simulink model "Assignment4"  (R2014a)
settings: Solver=FixedStepDiscrete  StartTime=0.0  StopTime=10.0  FixedStep=1  RelTol=1e-3
libraries: simulink x20, hdlsllib x20
settings Model: Creator=vu.du  LastModifiedBy=vu.du

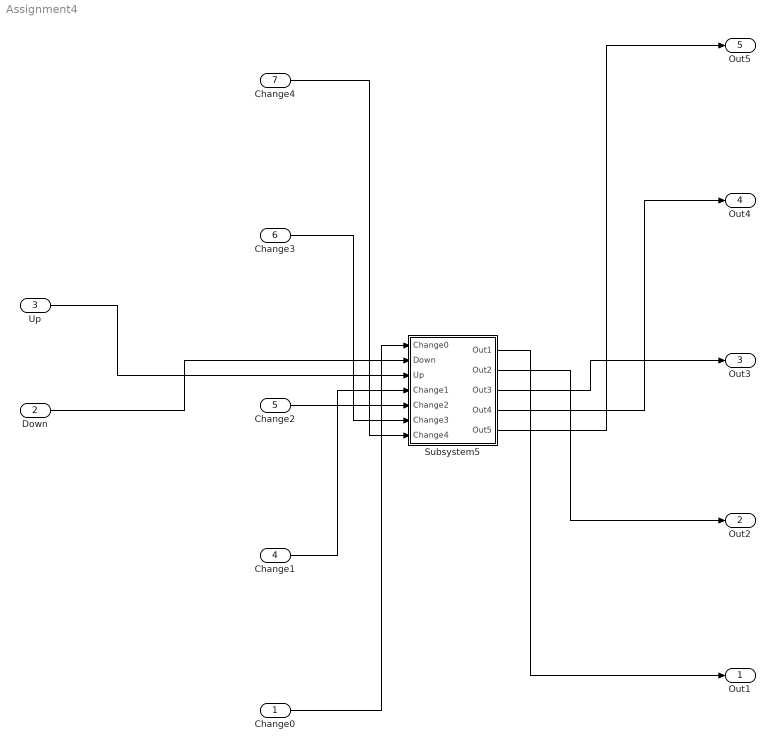
== system Assignment4 ==
  Change0 : Inport  OutDataTypeStr=boolean
  Down : Inport  Port=2  OutDataTypeStr=boolean
  Up : Inport  Port=3  OutDataTypeStr=boolean
  Change1 : Inport  Port=4  OutDataTypeStr=boolean
  Change2 : Inport  Port=5  OutDataTypeStr=boolean
  Change3 : Inport  Port=6  OutDataTypeStr=boolean
  Change4 : Inport  Port=7  OutDataTypeStr=boolean
  Subsystem5 : Subsystem  TreatAsAtomicUnit=on
  Out1 : Outport
  Out2 : Outport  Port=2
  Out3 : Outport  Port=3
  Out4 : Outport  Port=4
  Out5 : Outport  Port=5
  wires:
  Change0/1 -> Subsystem5/1(Change0)
  Down/1 -> Subsystem5/2(Down)
  Up/1 -> Subsystem5/3(Up)
  Change1/1 -> Subsystem5/4(Change1)
  Change2/1 -> Subsystem5/5(Change2)
  Change3/1 -> Subsystem5/6(Change3)
  Change4/1 -> Subsystem5/7(Change4)
  Subsystem5/1(Out1) -> Out1/1
  Subsystem5/2(Out2) -> Out2/1
  Subsystem5/3(Out3) -> Out3/1
  Subsystem5/4(Out4) -> Out4/1
  Subsystem5/5(Out5) -> Out5/1

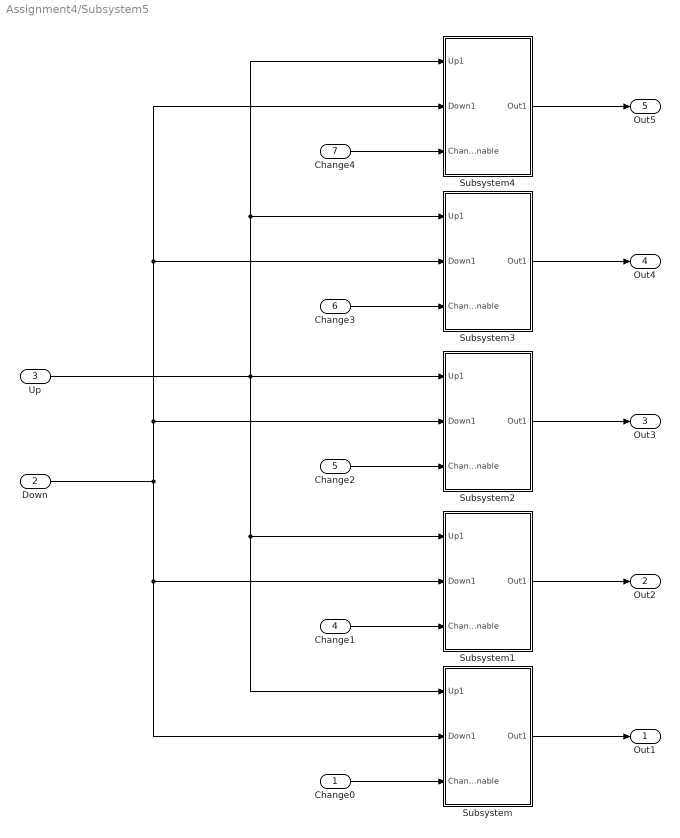
== system Assignment4/Subsystem5 ==
  Change0 : Inport  OutDataTypeStr=boolean
  Down : Inport  Port=2  OutDataTypeStr=boolean
  Up : Inport  Port=3  OutDataTypeStr=boolean
  Change1 : Inport  Port=4  OutDataTypeStr=boolean
  Change2 : Inport  Port=5  OutDataTypeStr=boolean
  Change3 : Inport  Port=6  OutDataTypeStr=boolean
  Change4 : Inport  Port=7  OutDataTypeStr=boolean
  Subsystem : Subsystem
  Subsystem1 : Subsystem
  Subsystem2 : Subsystem
  Subsystem3 : Subsystem
  Subsystem4 : Subsystem
  Out1 : Outport
  Out2 : Outport  Port=2
  Out3 : Outport  Port=3
  Out4 : Outport  Port=4
  Out5 : Outport  Port=5
  wires:
  Subsystem/1(Out1) -> Out1/1
  Subsystem4/1(Out1) -> Out5/1
  Change4/1 -> Subsystem4/3(ChangeEnable)
  Change1/1 -> Subsystem1/3(ChangeEnable)
  Down/1 -> Subsystem2/2(Down1), Subsystem3/2(Down1), Subsystem4/2(Down1), Subsystem/2(Down1), Subsystem1/2(Down1)
  Change0/1 -> Subsystem/3(ChangeEnable)
  Change3/1 -> Subsystem3/3(ChangeEnable)
  Change2/1 -> Subsystem2/3(ChangeEnable)
  Subsystem2/1(Out1) -> Out3/1
  Up/1 -> Subsystem1/1(Up1), Subsystem/1(Up1), Subsystem2/1(Up1), Subsystem3/1(Up1), Subsystem4/1(Up1)
  Subsystem1/1(Out1) -> Out2/1
  Subsystem3/1(Out1) -> Out4/1

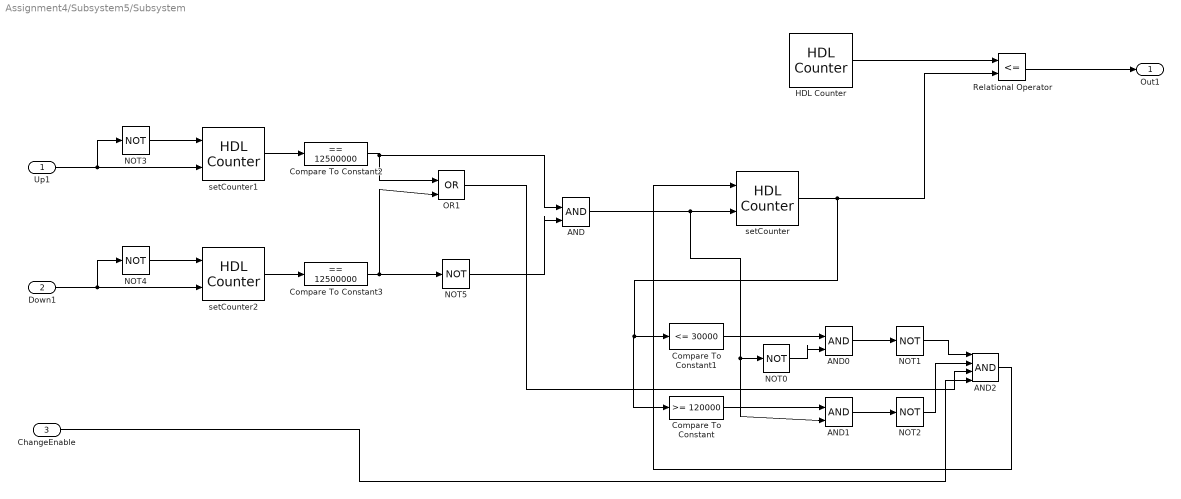
== system Assignment4/Subsystem5/Subsystem ==
  Up1 : Inport
  Down1 : Inport  Port=2
  ChangeEnable : Inport  Port=3
  AND : Logic  IconShape=distinctive  AllPortsSameDT=off  OutDataTypeStr=boolean
  AND0 : Logic  IconShape=distinctive  AllPortsSameDT=off  OutDataTypeStr=boolean
  AND1 : Logic  IconShape=distinctive  AllPortsSameDT=off  OutDataTypeStr=boolean
  AND2 : Logic  Inputs=4  IconShape=distinctive  AllPortsSameDT=off  OutDataTypeStr=boolean
  Compare To Constant : simulink/Logic and Bit Operations/Compare To Constant  relop=>=  const=120000  OutDataTypeStr=boolean
  Compare To Constant1 : simulink/Logic and Bit Operations/Compare To Constant  relop=<=  const=30000  OutDataTypeStr=boolean
  Compare To Constant2 : simulink/Logic and Bit Operations/Compare To Constant  relop===  const=12500000  OutDataTypeStr=boolean
  Compare To Constant3 : simulink/Logic and Bit Operations/Compare To Constant  relop===  const=12500000  OutDataTypeStr=boolean
  HDL Counter : hdlsllib/HDL Operations/HDL Counter  CountType=Count limited  CountInit=0  CountStep=1  CountMax=1000000  CountFromType=Initial value  CountFrom=0  CountResetPort=off  CountLoadPort=off  CountEnbPort=off  CountDirPort=off  CountDataType=Unsigned  CountWordLen=32  CountFracLen=0  CountSampTime=1
  NOT{0..5} (6 alike) : Logic  Operator=NOT  IconShape=distinctive  AllPortsSameDT=off  OutDataTypeStr=boolean
  OR1 : Logic  Operator=OR  IconShape=distinctive  AllPortsSameDT=off  OutDataTypeStr=boolean
  Relational Operator : RelationalOperator  Operator=<=  OutDataTypeStr=boolean
  setCounter : hdlsllib/HDL Operations/HDL Counter  CountType=Count limited  CountInit=75000  CountStep=6000  CountMax=120000  CountFromType=Specify  CountFrom=30000  CountResetPort=off  CountLoadPort=off  CountEnbPort=on  CountDirPort=on  CountDataType=Unsigned  CountWordLen=32  CountFracLen=0  CountSampTime=1
  setCounter1 : hdlsllib/HDL Operations/HDL Counter  CountType=Count limited  CountInit=0  CountStep=1  CountMax=50000000  CountFromType=Initial value  CountFrom=0  CountResetPort=on  CountLoadPort=off  CountEnbPort=on  CountDirPort=off  CountDataType=Unsigned  CountWordLen=32  CountFracLen=0  CountSampTime=1
  setCounter2 : hdlsllib/HDL Operations/HDL Counter  CountType=Count limited  CountInit=0  CountStep=1  CountMax=50000000  CountFromType=Initial value  CountFrom=0  CountResetPort=on  CountLoadPort=off  CountEnbPort=on  CountDirPort=off  CountDataType=Unsigned  CountWordLen=32  CountFracLen=0  CountSampTime=1
  Out1 : Outport
  wires:
  ChangeEnable/1 -> AND2/4
  Up1/1 -> setCounter1/2, NOT3/1
  Compare To Constant1/1 -> AND0/1
  NOT0/1 -> AND0/2
  AND2/1 -> setCounter/1
  Compare To Constant/1 -> AND1/1
  NOT1/1 -> AND2/1
  AND0/1 -> NOT1/1
  AND1/1 -> NOT2/1
  AND/1 -> AND1/2, NOT0/1, setCounter/2
  NOT2/1 -> AND2/2
  Relational Operator/1 -> Out1/1
  setCounter/1 -> Compare To Constant/1, Compare To Constant1/1, Relational Operator/2
  HDL Counter/1 -> Relational Operator/1
  Down1/1 -> setCounter2/2, NOT4/1
  NOT4/1 -> setCounter2/1
  setCounter2/1 -> Compare To Constant3/1
  Compare To Constant3/1 -> NOT5/1, OR1/2
  OR1/1 -> AND2/3
  setCounter1/1 -> Compare To Constant2/1
  Compare To Constant2/1 -> AND/1, OR1/1
  NOT3/1 -> setCounter1/1
  NOT5/1 -> AND/2

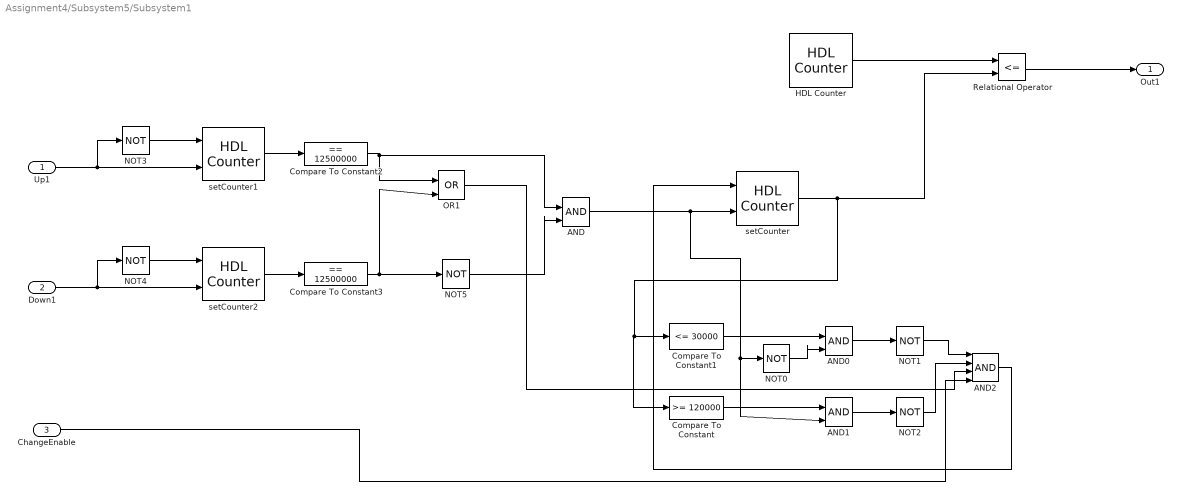
== system Assignment4/Subsystem5/Subsystem1 ==
  Up1 : Inport
  Down1 : Inport  Port=2
  ChangeEnable : Inport  Port=3
  AND : Logic  IconShape=distinctive  AllPortsSameDT=off  OutDataTypeStr=boolean
  AND0 : Logic  IconShape=distinctive  AllPortsSameDT=off  OutDataTypeStr=boolean
  AND1 : Logic  IconShape=distinctive  AllPortsSameDT=off  OutDataTypeStr=boolean
  AND2 : Logic  Inputs=4  IconShape=distinctive  AllPortsSameDT=off  OutDataTypeStr=boolean
  Compare To Constant : simulink/Logic and Bit Operations/Compare To Constant  relop=>=  const=120000  OutDataTypeStr=boolean
  Compare To Constant1 : simulink/Logic and Bit Operations/Compare To Constant  relop=<=  const=30000  OutDataTypeStr=boolean
  Compare To Constant2 : simulink/Logic and Bit Operations/Compare To Constant  relop===  const=12500000  OutDataTypeStr=boolean
  Compare To Constant3 : simulink/Logic and Bit Operations/Compare To Constant  relop===  const=12500000  OutDataTypeStr=boolean
  HDL Counter : hdlsllib/HDL Operations/HDL Counter  CountType=Count limited  CountInit=0  CountStep=1  CountMax=1000000  CountFromType=Initial value  CountFrom=0  CountResetPort=off  CountLoadPort=off  CountEnbPort=off  CountDirPort=off  CountDataType=Unsigned  CountWordLen=32  CountFracLen=0  CountSampTime=1
  NOT{0..5} (6 alike) : Logic  Operator=NOT  IconShape=distinctive  AllPortsSameDT=off  OutDataTypeStr=boolean
  OR1 : Logic  Operator=OR  IconShape=distinctive  AllPortsSameDT=off  OutDataTypeStr=boolean
  Relational Operator : RelationalOperator  Operator=<=  OutDataTypeStr=boolean
  setCounter : hdlsllib/HDL Operations/HDL Counter  CountType=Count limited  CountInit=75000  CountStep=6000  CountMax=120000  CountFromType=Specify  CountFrom=30000  CountResetPort=off  CountLoadPort=off  CountEnbPort=on  CountDirPort=on  CountDataType=Unsigned  CountWordLen=32  CountFracLen=0  CountSampTime=1
  setCounter1 : hdlsllib/HDL Operations/HDL Counter  CountType=Count limited  CountInit=0  CountStep=1  CountMax=50000000  CountFromType=Initial value  CountFrom=0  CountResetPort=on  CountLoadPort=off  CountEnbPort=on  CountDirPort=off  CountDataType=Unsigned  CountWordLen=32  CountFracLen=0  CountSampTime=1
  setCounter2 : hdlsllib/HDL Operations/HDL Counter  CountType=Count limited  CountInit=0  CountStep=1  CountMax=50000000  CountFromType=Initial value  CountFrom=0  CountResetPort=on  CountLoadPort=off  CountEnbPort=on  CountDirPort=off  CountDataType=Unsigned  CountWordLen=32  CountFracLen=0  CountSampTime=1
  Out1 : Outport
  wires:
  ChangeEnable/1 -> AND2/4
  Up1/1 -> setCounter1/2, NOT3/1
  Compare To Constant1/1 -> AND0/1
  NOT0/1 -> AND0/2
  AND2/1 -> setCounter/1
  Compare To Constant/1 -> AND1/1
  NOT1/1 -> AND2/1
  AND0/1 -> NOT1/1
  AND1/1 -> NOT2/1
  AND/1 -> AND1/2, NOT0/1, setCounter/2
  NOT2/1 -> AND2/2
  Relational Operator/1 -> Out1/1
  setCounter/1 -> Compare To Constant/1, Compare To Constant1/1, Relational Operator/2
  HDL Counter/1 -> Relational Operator/1
  Down1/1 -> setCounter2/2, NOT4/1
  NOT4/1 -> setCounter2/1
  setCounter2/1 -> Compare To Constant3/1
  Compare To Constant3/1 -> NOT5/1, OR1/2
  OR1/1 -> AND2/3
  setCounter1/1 -> Compare To Constant2/1
  Compare To Constant2/1 -> AND/1, OR1/1
  NOT3/1 -> setCounter1/1
  NOT5/1 -> AND/2

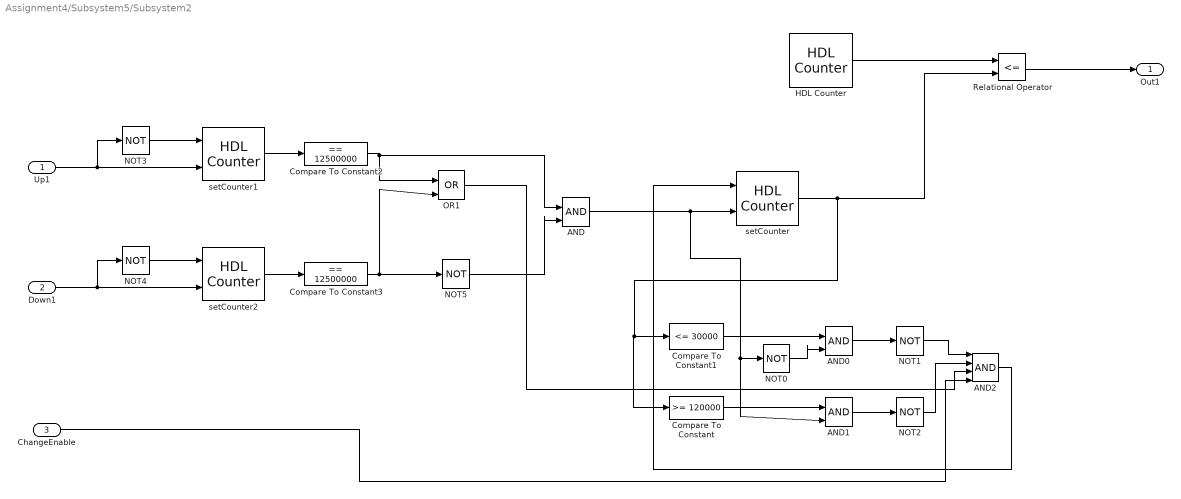
== system Assignment4/Subsystem5/Subsystem2 ==
  Up1 : Inport
  Down1 : Inport  Port=2
  ChangeEnable : Inport  Port=3
  AND : Logic  IconShape=distinctive  AllPortsSameDT=off  OutDataTypeStr=boolean
  AND0 : Logic  IconShape=distinctive  AllPortsSameDT=off  OutDataTypeStr=boolean
  AND1 : Logic  IconShape=distinctive  AllPortsSameDT=off  OutDataTypeStr=boolean
  AND2 : Logic  Inputs=4  IconShape=distinctive  AllPortsSameDT=off  OutDataTypeStr=boolean
  Compare To Constant : simulink/Logic and Bit Operations/Compare To Constant  relop=>=  const=120000  OutDataTypeStr=boolean
  Compare To Constant1 : simulink/Logic and Bit Operations/Compare To Constant  relop=<=  const=30000  OutDataTypeStr=boolean
  Compare To Constant2 : simulink/Logic and Bit Operations/Compare To Constant  relop===  const=12500000  OutDataTypeStr=boolean
  Compare To Constant3 : simulink/Logic and Bit Operations/Compare To Constant  relop===  const=12500000  OutDataTypeStr=boolean
  HDL Counter : hdlsllib/HDL Operations/HDL Counter  CountType=Count limited  CountInit=0  CountStep=1  CountMax=1000000  CountFromType=Initial value  CountFrom=0  CountResetPort=off  CountLoadPort=off  CountEnbPort=off  CountDirPort=off  CountDataType=Unsigned  CountWordLen=32  CountFracLen=0  CountSampTime=1
  NOT{0..5} (6 alike) : Logic  Operator=NOT  IconShape=distinctive  AllPortsSameDT=off  OutDataTypeStr=boolean
  OR1 : Logic  Operator=OR  IconShape=distinctive  AllPortsSameDT=off  OutDataTypeStr=boolean
  Relational Operator : RelationalOperator  Operator=<=  OutDataTypeStr=boolean
  setCounter : hdlsllib/HDL Operations/HDL Counter  CountType=Count limited  CountInit=75000  CountStep=6000  CountMax=120000  CountFromType=Specify  CountFrom=30000  CountResetPort=off  CountLoadPort=off  CountEnbPort=on  CountDirPort=on  CountDataType=Unsigned  CountWordLen=32  CountFracLen=0  CountSampTime=1
  setCounter1 : hdlsllib/HDL Operations/HDL Counter  CountType=Count limited  CountInit=0  CountStep=1  CountMax=50000000  CountFromType=Initial value  CountFrom=0  CountResetPort=on  CountLoadPort=off  CountEnbPort=on  CountDirPort=off  CountDataType=Unsigned  CountWordLen=32  CountFracLen=0  CountSampTime=1
  setCounter2 : hdlsllib/HDL Operations/HDL Counter  CountType=Count limited  CountInit=0  CountStep=1  CountMax=50000000  CountFromType=Initial value  CountFrom=0  CountResetPort=on  CountLoadPort=off  CountEnbPort=on  CountDirPort=off  CountDataType=Unsigned  CountWordLen=32  CountFracLen=0  CountSampTime=1
  Out1 : Outport
  wires:
  ChangeEnable/1 -> AND2/4
  Up1/1 -> setCounter1/2, NOT3/1
  Compare To Constant1/1 -> AND0/1
  NOT0/1 -> AND0/2
  AND2/1 -> setCounter/1
  Compare To Constant/1 -> AND1/1
  NOT1/1 -> AND2/1
  AND0/1 -> NOT1/1
  AND1/1 -> NOT2/1
  AND/1 -> AND1/2, NOT0/1, setCounter/2
  NOT2/1 -> AND2/2
  Relational Operator/1 -> Out1/1
  setCounter/1 -> Compare To Constant/1, Compare To Constant1/1, Relational Operator/2
  HDL Counter/1 -> Relational Operator/1
  Down1/1 -> setCounter2/2, NOT4/1
  NOT4/1 -> setCounter2/1
  setCounter2/1 -> Compare To Constant3/1
  Compare To Constant3/1 -> NOT5/1, OR1/2
  OR1/1 -> AND2/3
  setCounter1/1 -> Compare To Constant2/1
  Compare To Constant2/1 -> AND/1, OR1/1
  NOT3/1 -> setCounter1/1
  NOT5/1 -> AND/2

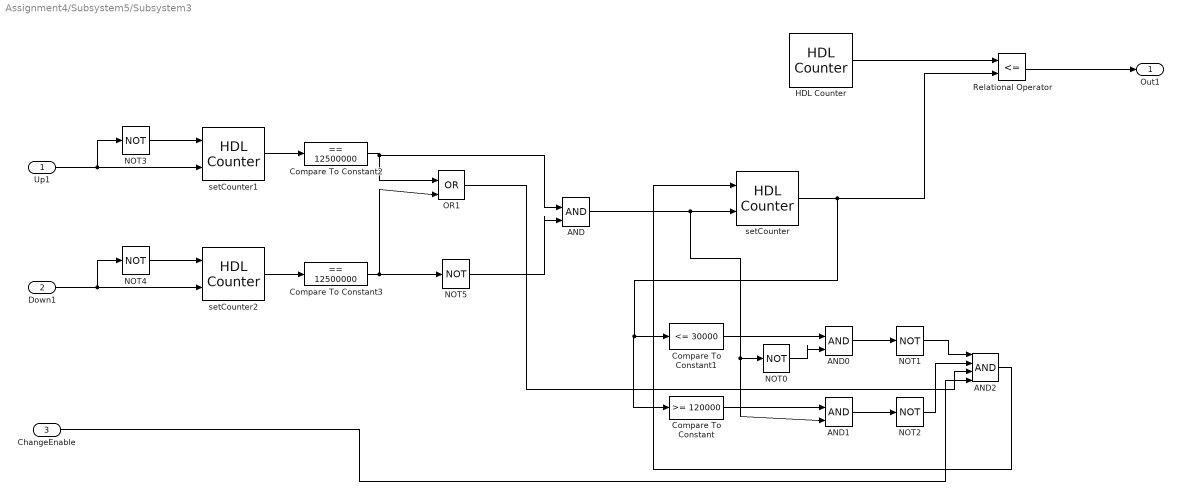
== system Assignment4/Subsystem5/Subsystem3 ==
  Up1 : Inport
  Down1 : Inport  Port=2
  ChangeEnable : Inport  Port=3
  AND : Logic  IconShape=distinctive  AllPortsSameDT=off  OutDataTypeStr=boolean
  AND0 : Logic  IconShape=distinctive  AllPortsSameDT=off  OutDataTypeStr=boolean
  AND1 : Logic  IconShape=distinctive  AllPortsSameDT=off  OutDataTypeStr=boolean
  AND2 : Logic  Inputs=4  IconShape=distinctive  AllPortsSameDT=off  OutDataTypeStr=boolean
  Compare To Constant : simulink/Logic and Bit Operations/Compare To Constant  relop=>=  const=120000  OutDataTypeStr=boolean
  Compare To Constant1 : simulink/Logic and Bit Operations/Compare To Constant  relop=<=  const=30000  OutDataTypeStr=boolean
  Compare To Constant2 : simulink/Logic and Bit Operations/Compare To Constant  relop===  const=12500000  OutDataTypeStr=boolean
  Compare To Constant3 : simulink/Logic and Bit Operations/Compare To Constant  relop===  const=12500000  OutDataTypeStr=boolean
  HDL Counter : hdlsllib/HDL Operations/HDL Counter  CountType=Count limited  CountInit=0  CountStep=1  CountMax=1000000  CountFromType=Initial value  CountFrom=0  CountResetPort=off  CountLoadPort=off  CountEnbPort=off  CountDirPort=off  CountDataType=Unsigned  CountWordLen=32  CountFracLen=0  CountSampTime=1
  NOT{0..5} (6 alike) : Logic  Operator=NOT  IconShape=distinctive  AllPortsSameDT=off  OutDataTypeStr=boolean
  OR1 : Logic  Operator=OR  IconShape=distinctive  AllPortsSameDT=off  OutDataTypeStr=boolean
  Relational Operator : RelationalOperator  Operator=<=  OutDataTypeStr=boolean
  setCounter : hdlsllib/HDL Operations/HDL Counter  CountType=Count limited  CountInit=75000  CountStep=6000  CountMax=120000  CountFromType=Specify  CountFrom=30000  CountResetPort=off  CountLoadPort=off  CountEnbPort=on  CountDirPort=on  CountDataType=Unsigned  CountWordLen=32  CountFracLen=0  CountSampTime=1
  setCounter1 : hdlsllib/HDL Operations/HDL Counter  CountType=Count limited  CountInit=0  CountStep=1  CountMax=50000000  CountFromType=Initial value  CountFrom=0  CountResetPort=on  CountLoadPort=off  CountEnbPort=on  CountDirPort=off  CountDataType=Unsigned  CountWordLen=32  CountFracLen=0  CountSampTime=1
  setCounter2 : hdlsllib/HDL Operations/HDL Counter  CountType=Count limited  CountInit=0  CountStep=1  CountMax=50000000  CountFromType=Initial value  CountFrom=0  CountResetPort=on  CountLoadPort=off  CountEnbPort=on  CountDirPort=off  CountDataType=Unsigned  CountWordLen=32  CountFracLen=0  CountSampTime=1
  Out1 : Outport
  wires:
  ChangeEnable/1 -> AND2/4
  Up1/1 -> setCounter1/2, NOT3/1
  Compare To Constant1/1 -> AND0/1
  NOT0/1 -> AND0/2
  AND2/1 -> setCounter/1
  Compare To Constant/1 -> AND1/1
  NOT1/1 -> AND2/1
  AND0/1 -> NOT1/1
  AND1/1 -> NOT2/1
  AND/1 -> AND1/2, NOT0/1, setCounter/2
  NOT2/1 -> AND2/2
  Relational Operator/1 -> Out1/1
  setCounter/1 -> Compare To Constant/1, Compare To Constant1/1, Relational Operator/2
  HDL Counter/1 -> Relational Operator/1
  Down1/1 -> setCounter2/2, NOT4/1
  NOT4/1 -> setCounter2/1
  setCounter2/1 -> Compare To Constant3/1
  Compare To Constant3/1 -> NOT5/1, OR1/2
  OR1/1 -> AND2/3
  setCounter1/1 -> Compare To Constant2/1
  Compare To Constant2/1 -> AND/1, OR1/1
  NOT3/1 -> setCounter1/1
  NOT5/1 -> AND/2

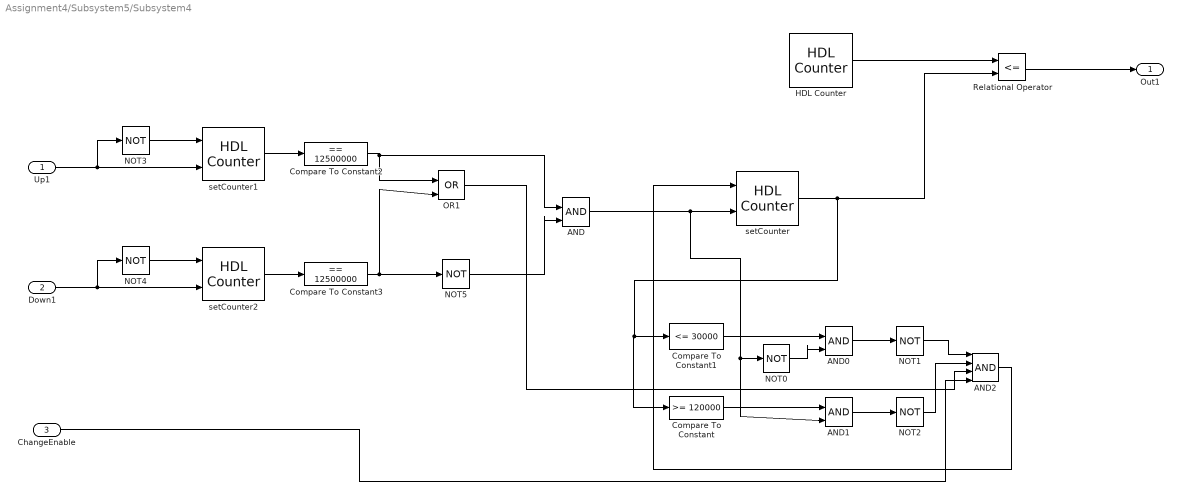
== system Assignment4/Subsystem5/Subsystem4 ==
  Up1 : Inport
  Down1 : Inport  Port=2
  ChangeEnable : Inport  Port=3
  AND : Logic  IconShape=distinctive  AllPortsSameDT=off  OutDataTypeStr=boolean
  AND0 : Logic  IconShape=distinctive  AllPortsSameDT=off  OutDataTypeStr=boolean
  AND1 : Logic  IconShape=distinctive  AllPortsSameDT=off  OutDataTypeStr=boolean
  AND2 : Logic  Inputs=4  IconShape=distinctive  AllPortsSameDT=off  OutDataTypeStr=boolean
  Compare To Constant : simulink/Logic and Bit Operations/Compare To Constant  relop=>=  const=120000  OutDataTypeStr=boolean
  Compare To Constant1 : simulink/Logic and Bit Operations/Compare To Constant  relop=<=  const=30000  OutDataTypeStr=boolean
  Compare To Constant2 : simulink/Logic and Bit Operations/Compare To Constant  relop===  const=12500000  OutDataTypeStr=boolean
  Compare To Constant3 : simulink/Logic and Bit Operations/Compare To Constant  relop===  const=12500000  OutDataTypeStr=boolean
  HDL Counter : hdlsllib/HDL Operations/HDL Counter  CountType=Count limited  CountInit=0  CountStep=1  CountMax=1000000  CountFromType=Initial value  CountFrom=0  CountResetPort=off  CountLoadPort=off  CountEnbPort=off  CountDirPort=off  CountDataType=Unsigned  CountWordLen=32  CountFracLen=0  CountSampTime=1
  NOT{0..5} (6 alike) : Logic  Operator=NOT  IconShape=distinctive  AllPortsSameDT=off  OutDataTypeStr=boolean
  OR1 : Logic  Operator=OR  IconShape=distinctive  AllPortsSameDT=off  OutDataTypeStr=boolean
  Relational Operator : RelationalOperator  Operator=<=  OutDataTypeStr=boolean
  setCounter : hdlsllib/HDL Operations/HDL Counter  CountType=Count limited  CountInit=75000  CountStep=6000  CountMax=120000  CountFromType=Specify  CountFrom=30000  CountResetPort=off  CountLoadPort=off  CountEnbPort=on  CountDirPort=on  CountDataType=Unsigned  CountWordLen=32  CountFracLen=0  CountSampTime=1
  setCounter1 : hdlsllib/HDL Operations/HDL Counter  CountType=Count limited  CountInit=0  CountStep=1  CountMax=50000000  CountFromType=Initial value  CountFrom=0  CountResetPort=on  CountLoadPort=off  CountEnbPort=on  CountDirPort=off  CountDataType=Unsigned  CountWordLen=32  CountFracLen=0  CountSampTime=1
  setCounter2 : hdlsllib/HDL Operations/HDL Counter  CountType=Count limited  CountInit=0  CountStep=1  CountMax=50000000  CountFromType=Initial value  CountFrom=0  CountResetPort=on  CountLoadPort=off  CountEnbPort=on  CountDirPort=off  CountDataType=Unsigned  CountWordLen=32  CountFracLen=0  CountSampTime=1
  Out1 : Outport
  wires:
  ChangeEnable/1 -> AND2/4
  Up1/1 -> setCounter1/2, NOT3/1
  Compare To Constant1/1 -> AND0/1
  NOT0/1 -> AND0/2
  AND2/1 -> setCounter/1
  Compare To Constant/1 -> AND1/1
  NOT1/1 -> AND2/1
  AND0/1 -> NOT1/1
  AND1/1 -> NOT2/1
  AND/1 -> AND1/2, NOT0/1, setCounter/2
  NOT2/1 -> AND2/2
  Relational Operator/1 -> Out1/1
  setCounter/1 -> Compare To Constant/1, Compare To Constant1/1, Relational Operator/2
  HDL Counter/1 -> Relational Operator/1
  Down1/1 -> setCounter2/2, NOT4/1
  NOT4/1 -> setCounter2/1
  setCounter2/1 -> Compare To Constant3/1
  Compare To Constant3/1 -> NOT5/1, OR1/2
  OR1/1 -> AND2/3
  setCounter1/1 -> Compare To Constant2/1
  Compare To Constant2/1 -> AND/1, OR1/1
  NOT3/1 -> setCounter1/1
  NOT5/1 -> AND/2
